simulink model "SIL_model"  (R2020a)
settings: Solver=ode4  StartTime=0.0  StopTime=30  FixedStep=0.001  RelTol=1e-3
InitFcn:
  | Init_control;
values from neighbouring files (symbols this model uses):
  layer1 = double(results{1,1}.layer9)    [load_parameter.m]
  layer2 = double(results{1,1}.layer10)    [load_parameter.m]
  layer3 = double(results{1,1}.layer11)    [load_parameter.m]
  layer4 = double(results{1,1}.layer12)    [load_parameter.m]
  layer5 = double(results{1,1}.layer13)    [load_parameter.m]
  layer6 = double(results{1,1}.layer14)    [load_parameter.m]
  std = sqrt(max(a,0.01))    [load_parameter.m]
undefined symbols (not defined in the file or in its folder): DWORK0, DWORK1, DWORK10, DWORK11, DWORK12, DWORK13, DWORK14, DWORK15, DWORK2, DWORK3, DWORK4, DWORK5, DWORK6, DWORK7, DWORK8, DWORK9, earthRadius, KiPitchAttitude, KiRollAttitude, Kp_RP_ANGLE, MAX_CONTROL_ANGLE_RATE_Y, MAX_CONTROL_ANGLE_RP, ModelInit_RPM, ModelParam_envAltitude, ModelParam_GlobalNoiseGainSwitch, ModelParam_GPSLatLong, ModelParam_motorCr, ModelParam_motorJm, ModelParam_motorMinThr, ModelParam_motorT, ModelParam_motorWb, ModelParam_rotorCm, ModelParam_rotorCt, ModelParam_uavCCm, ModelParam_uavCd, ModelParam_uavDearo, ModelParam_uavJ, ModelParam_uavMass, ModelParam_uavR, ModelParam_uavType, Receive, Send
libraries: aerolibfltsims x4, simulink x2, shared6dof x1, aerolibanimutils x1
(part 2 of 2)

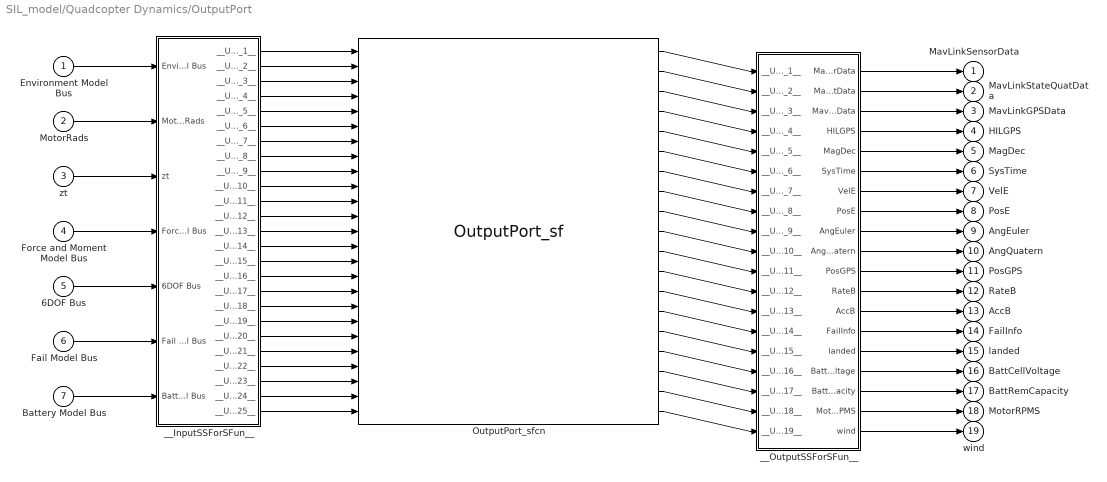
== system SIL_model/Quadcopter Dynamics/OutputPort ==
  Environment Model Bus : Inport
  MotorRads : Inport  Port=2
  zt : Inport  Port=3
  Force and Moment Model Bus : Inport  Port=4
  6DOF Bus : Inport  Port=5
  Fail Model Bus : Inport  Port=6
  Battery Model Bus : Inport  Port=7
  OutputPort_sfcn : S-Function  FunctionName=OutputPort_sf  Parameters=sfcnParam1, sfcnParam2, sfcnParam3  SFunctionModules=""  SFunctionDeploymentMode=off  EnableBusSupport=off  SFcnStateName=DWORK0,DWORK1,DWORK2,DWORK3,DWORK4,DWORK5,DWORK6,DWORK7,DWORK8,DWORK9  mask{rtw_sf_name=OutputPort_sf, showVar=off, sfcnParam1=sfcnParam1, sfcnParam2=sfcnParam2, sfcnParam3=sfcnParam3}
      mask prompts: rtw_sf_name "Simulink:masks:GenSFuncName_MP"; showVar "Simulink:masks:GenSFuncShowModuleList_MP"; sfcnParam1 "ModelParam_GPSLatLong:"; sfcnParam2 "ModelParam_GlobalNoiseGainSwitch:"; sfcnParam3 "ModelParam_envAltitude:"
      mask help: Simulink:masks:GenSFuncDesc_MD
      mask init: same as SIL_model/Quadcopter Dynamics/Battery Model/Battery Model_sfcn
      settings: SFcnIsStateOwnerBlock=on
      settings: CopyFcn=|
      | if ~strcmp(get_param(gcb,'Linkstatus'),'none') && ...
      | ~strcmp(get_param(gcb,'Linkstatus'),'implicit')
      |   set_param(gcb,'LinkStatus','none');
      | end
      mask Help: eval('feval(''rtwprivate'',''rtwhelpview'',''rtw_sfcn_block'')');
      mask Display:
      | port_label('input',1,'PosGPS');
      | port_label('input',2,'gravity');
      | port_label('input',3,'TempC');
      | port_label('input',4,'AirPressure');
      | port_label('input',5,'Rho');
      | port_label('input',6,'Windb');
      | port_label('input',7,'Wind');
      | port_label('input',8,'MotorRads');
      | port_label('input',9,'zt');
      | port_label('input',10,'Fb');
      | port_label('input',11,'Mb');
      | port_label('input',12,'landed');
      | port_label('input',13,'Ve');
      | port_label('input',14,'Xe');
      | port_label('input',15,'Eular(rad)');
      | port_label('input',16,'DCM');
      | port_label('input',17,'Vb');
      | port_label('input',18,'wb');
      | port_label('input',19,'dwb/dt');
      | port_label('input',20,'m');
      | port_label('input',21,'J');
      | port_label('input',22,'dM');
      | port_label('input',23,'PWMOut');
      | port_label('input',24,'cellVol');
      | port_label('input',25,'remCapa');
      | port_label('output',1,'MavLinkSensorData');
      | port_label('output',2,'MavLinkStateQuatData');
      | port_label('output',3,'MavLinkGPSData');
      | port_label('output',4,'HILGPS');
      | port_label('output',5,'MagDec');
      | port_label('output',6,'SysTime');
      | port_label('output',7,'VelE');
      | port_label('output',8,'PosE');
      | port_label('output',9,'AngEuler');
      | port_label('output',10,'AngQuatern');
      | port_label('output',11,'PosGPSb');
      | port_label('output',12,'RateB');
      | port_label('output',13,'AccB');
      | port_label('output',14,'FailInfo');
      | port_label('output',15,'landedb');
      | port_label('output',16,'BattCellVoltage');
      | port_label('output',17,'BattRemCapacity');
      | port_label('output',18,'MotorRPMS');
      | port_label('output',19,'wind');
  __InputSSForSFun__ : Subsystem
  __OutputSSForSFun__ : Subsystem
  MavLinkSensorData : Outport  OutDataTypeStr=Bus: MavLinkSensor  SampleTime=[-1 0]  VectorParamsAs1DForOutWhenUnconnected=off  BusOutputAsStruct=on
  MavLinkStateQuatData : Outport  Port=2  OutDataTypeStr=Bus: MavLinkStateQuat  SampleTime=[-1 0]  VectorParamsAs1DForOutWhenUnconnected=off  BusOutputAsStruct=on
  MavLinkGPSData : Outport  Port=3  OutDataTypeStr=Bus: MavLinkGPS  SampleTime=[-1 0]  VectorParamsAs1DForOutWhenUnconnected=off  BusOutputAsStruct=on
  HILGPS : Outport  Port=4  OutDataTypeStr=Bus: HILGPS  SampleTime=[-1 0]  VectorParamsAs1DForOutWhenUnconnected=off  BusOutputAsStruct=on
  MagDec : Outport  Port=5  VectorParamsAs1DForOutWhenUnconnected=off
  SysTime : Outport  Port=6  VectorParamsAs1DForOutWhenUnconnected=off
  VelE : Outport  Port=7  VectorParamsAs1DForOutWhenUnconnected=off
  PosE : Outport  Port=8  VectorParamsAs1DForOutWhenUnconnected=off
  AngEuler : Outport  Port=9  VectorParamsAs1DForOutWhenUnconnected=off
  AngQuatern : Outport  Port=10  VectorParamsAs1DForOutWhenUnconnected=off
  PosGPS : Outport  Port=11  VectorParamsAs1DForOutWhenUnconnected=off
  RateB : Outport  Port=12  VectorParamsAs1DForOutWhenUnconnected=off
  AccB : Outport  Port=13  VectorParamsAs1DForOutWhenUnconnected=off
  FailInfo : Outport  Port=14  VectorParamsAs1DForOutWhenUnconnected=off
  landed : Outport  Port=15  VectorParamsAs1DForOutWhenUnconnected=off
  BattCellVoltage : Outport  Port=16  VectorParamsAs1DForOutWhenUnconnected=off
  BattRemCapacity : Outport  Port=17  VectorParamsAs1DForOutWhenUnconnected=off
  MotorRPMS : Outport  Port=18  VectorParamsAs1DForOutWhenUnconnected=off
  wind : Outport  Port=19  VectorParamsAs1DForOutWhenUnconnected=off
  wires:
  Environment Model Bus/1 -> __InputSSForSFun__/1(Environment Model Bus)
  MotorRads/1 -> __InputSSForSFun__/2(MotorRads)
  zt/1 -> __InputSSForSFun__/3(zt)
  Force and Moment Model Bus/1 -> __InputSSForSFun__/4(Force and Moment Model Bus)
  6DOF Bus/1 -> __InputSSForSFun__/5(6DOF Bus)
  Fail Model Bus/1 -> __InputSSForSFun__/6(Fail Model Bus)
  Battery Model Bus/1 -> __InputSSForSFun__/7(Battery Model Bus)
  __InputSSForSFun__/1(__UniqueOutportName__1__) -> OutputPort_sfcn/1
  __InputSSForSFun__/2(__UniqueOutportName__2__) -> OutputPort_sfcn/2
  __InputSSForSFun__/3(__UniqueOutportName__3__) -> OutputPort_sfcn/3
  __InputSSForSFun__/4(__UniqueOutportName__4__) -> OutputPort_sfcn/4
  __InputSSForSFun__/5(__UniqueOutportName__5__) -> OutputPort_sfcn/5
  __InputSSForSFun__/6(__UniqueOutportName__6__) -> OutputPort_sfcn/6
  __InputSSForSFun__/7(__UniqueOutportName__7__) -> OutputPort_sfcn/7
  __InputSSForSFun__/8(__UniqueOutportName__8__) -> OutputPort_sfcn/8
  __InputSSForSFun__/9(__UniqueOutportName__9__) -> OutputPort_sfcn/9
  __InputSSForSFun__/10(__UniqueOutportName__10__) -> OutputPort_sfcn/10
  __InputSSForSFun__/11(__UniqueOutportName__11__) -> OutputPort_sfcn/11
  __InputSSForSFun__/12(__UniqueOutportName__12__) -> OutputPort_sfcn/12
  __InputSSForSFun__/13(__UniqueOutportName__13__) -> OutputPort_sfcn/13
  __InputSSForSFun__/14(__UniqueOutportName__14__) -> OutputPort_sfcn/14
  __InputSSForSFun__/15(__UniqueOutportName__15__) -> OutputPort_sfcn/15
  __InputSSForSFun__/16(__UniqueOutportName__16__) -> OutputPort_sfcn/16
  __InputSSForSFun__/17(__UniqueOutportName__17__) -> OutputPort_sfcn/17
  __InputSSForSFun__/18(__UniqueOutportName__18__) -> OutputPort_sfcn/18
  __InputSSForSFun__/19(__UniqueOutportName__19__) -> OutputPort_sfcn/19
  __InputSSForSFun__/20(__UniqueOutportName__20__) -> OutputPort_sfcn/20
  __InputSSForSFun__/21(__UniqueOutportName__21__) -> OutputPort_sfcn/21
  __InputSSForSFun__/22(__UniqueOutportName__22__) -> OutputPort_sfcn/22
  __InputSSForSFun__/23(__UniqueOutportName__23__) -> OutputPort_sfcn/23
  __InputSSForSFun__/24(__UniqueOutportName__24__) -> OutputPort_sfcn/24
  __InputSSForSFun__/25(__UniqueOutportName__25__) -> OutputPort_sfcn/25
  OutputPort_sfcn/1 -> __OutputSSForSFun__/1(__UniqueInportName__1__)
  OutputPort_sfcn/2 -> __OutputSSForSFun__/2(__UniqueInportName__2__)
  OutputPort_sfcn/3 -> __OutputSSForSFun__/3(__UniqueInportName__3__)
  OutputPort_sfcn/4 -> __OutputSSForSFun__/4(__UniqueInportName__4__)
  OutputPort_sfcn/5 -> __OutputSSForSFun__/5(__UniqueInportName__5__)
  OutputPort_sfcn/6 -> __OutputSSForSFun__/6(__UniqueInportName__6__)
  OutputPort_sfcn/7 -> __OutputSSForSFun__/7(__UniqueInportName__7__)
  OutputPort_sfcn/8 -> __OutputSSForSFun__/8(__UniqueInportName__8__)
  OutputPort_sfcn/9 -> __OutputSSForSFun__/9(__UniqueInportName__9__)
  OutputPort_sfcn/10 -> __OutputSSForSFun__/10(__UniqueInportName__10__)
  OutputPort_sfcn/11 -> __OutputSSForSFun__/11(__UniqueInportName__11__)
  OutputPort_sfcn/12 -> __OutputSSForSFun__/12(__UniqueInportName__12__)
  OutputPort_sfcn/13 -> __OutputSSForSFun__/13(__UniqueInportName__13__)
  OutputPort_sfcn/14 -> __OutputSSForSFun__/14(__UniqueInportName__14__)
  OutputPort_sfcn/15 -> __OutputSSForSFun__/15(__UniqueInportName__15__)
  OutputPort_sfcn/16 -> __OutputSSForSFun__/16(__UniqueInportName__16__)
  OutputPort_sfcn/17 -> __OutputSSForSFun__/17(__UniqueInportName__17__)
  OutputPort_sfcn/18 -> __OutputSSForSFun__/18(__UniqueInportName__18__)
  OutputPort_sfcn/19 -> __OutputSSForSFun__/19(__UniqueInportName__19__)
  __OutputSSForSFun__/1(MavLinkSensorData) -> MavLinkSensorData/1
  __OutputSSForSFun__/2(MavLinkStateQuatData) -> MavLinkStateQuatData/1
  __OutputSSForSFun__/3(MavLinkGPSData) -> MavLinkGPSData/1
  __OutputSSForSFun__/4(HILGPS) -> HILGPS/1
  __OutputSSForSFun__/5(MagDec) -> MagDec/1
  __OutputSSForSFun__/6(SysTime) -> SysTime/1
  __OutputSSForSFun__/7(VelE) -> VelE/1
  __OutputSSForSFun__/8(PosE) -> PosE/1
  __OutputSSForSFun__/9(AngEuler) -> AngEuler/1
  __OutputSSForSFun__/10(AngQuatern) -> AngQuatern/1
  __OutputSSForSFun__/11(PosGPS) -> PosGPS/1
  __OutputSSForSFun__/12(RateB) -> RateB/1
  __OutputSSForSFun__/13(AccB) -> AccB/1
  __OutputSSForSFun__/14(FailInfo) -> FailInfo/1
  __OutputSSForSFun__/15(landed) -> landed/1
  __OutputSSForSFun__/16(BattCellVoltage) -> BattCellVoltage/1
  __OutputSSForSFun__/17(BattRemCapacity) -> BattRemCapacity/1
  __OutputSSForSFun__/18(MotorRPMS) -> MotorRPMS/1
  __OutputSSForSFun__/19(wind) -> wind/1

== system SIL_model/Quadcopter Dynamics/Separation of float Data1 ==
  note: 小数部分
  float_Data : Inport
  Add2 : Sum  Inputs=+-
  Integer Uint : Constant  Value=IntUint
  Math Function1 : Math  Operator=mod  SignedPower=on  SaturateOnIntegerOverflow=on
  Integer_Part : Outport  VectorParamsAs1DForOutWhenUnconnected=off
  decimalt_Part : Outport  Port=2  VectorParamsAs1DForOutWhenUnconnected=off
  wires:
  Math Function1/1 -> decimalt_Part/1, Add2/2
  Integer Uint/1 -> Math Function1/2
  Add2/1 -> Integer_Part/1
  float_Data/1 -> Math Function1/1, Add2/1

== system SIL_model/Quadcopter Dynamics/Battery Model/__InputSSForSFun__ ==
  PWMin : Inport
  __UniqueOutportName__1__ : Outport  VectorParamsAs1DForOutWhenUnconnected=off
  wires:
  PWMin/1 -> __UniqueOutportName__1__/1

== system SIL_model/Quadcopter Dynamics/Battery Model/__OutputSSForSFun__ ==
  __UniqueInportName__1__ : Inport
  __UniqueInportName__2__ : Inport  Port=2
  __UniqueInportName__3__ : Inport  Port=3
  Mux1 : BusCreator  Inputs=3
  Battery Model Bus : Outport  VectorParamsAs1DForOutWhenUnconnected=off
  wires:
  __UniqueInportName__1__/1 -> Mux1/1  "PWMOut"
  __UniqueInportName__2__/1 -> Mux1/2  "cellVol"
  __UniqueInportName__3__/1 -> Mux1/3  "remCapa"
  Mux1/1 -> Battery Model Bus/1

== system SIL_model/Quadcopter Dynamics/Environment Model/__InputSSForSFun__ ==
  6DOF Bus : Inport
  temporaryBusSelectName_1 : BusSelector  OutputSignals=Ve,Xe,Eular(rad),DCM,Vb,wb,dwb/dt
  __UniqueOutportName__1__ : Outport  VectorParamsAs1DForOutWhenUnconnected=off
  __UniqueOutportName__2__ : Outport  Port=2  VectorParamsAs1DForOutWhenUnconnected=off
  __UniqueOutportName__3__ : Outport  Port=3  VectorParamsAs1DForOutWhenUnconnected=off
  __UniqueOutportName__4__ : Outport  Port=4  VectorParamsAs1DForOutWhenUnconnected=off
  __UniqueOutportName__5__ : Outport  Port=5  VectorParamsAs1DForOutWhenUnconnected=off
  __UniqueOutportName__6__ : Outport  Port=6  VectorParamsAs1DForOutWhenUnconnected=off
  __UniqueOutportName__7__ : Outport  Port=7  VectorParamsAs1DForOutWhenUnconnected=off
  wires:
  6DOF Bus/1 -> temporaryBusSelectName_1/1
  temporaryBusSelectName_1/1 -> __UniqueOutportName__1__/1  "<Ve>"
  temporaryBusSelectName_1/2 -> __UniqueOutportName__2__/1  "<Xe>"
  temporaryBusSelectName_1/3 -> __UniqueOutportName__3__/1  "<Eular(rad)>"
  temporaryBusSelectName_1/4 -> __UniqueOutportName__4__/1  "<DCM>"
  temporaryBusSelectName_1/5 -> __UniqueOutportName__5__/1  "<Vb>"
  temporaryBusSelectName_1/6 -> __UniqueOutportName__6__/1  "<wb>"
  temporaryBusSelectName_1/7 -> __UniqueOutportName__7__/1  "<dwb/dt>"

== system SIL_model/Quadcopter Dynamics/Environment Model/__OutputSSForSFun__ ==
  __UniqueInportName__1__ : Inport
  __UniqueInportName__2__ : Inport  Port=2
  __UniqueInportName__3__ : Inport  Port=3
  __UniqueInportName__4__ : Inport  Port=4
  __UniqueInportName__5__ : Inport  Port=5
  __UniqueInportName__6__ : Inport  Port=6
  __UniqueInportName__7__ : Inport  Port=7
  Mux1 : BusCreator  Inputs=7
  Environment Model Bus : Outport  VectorParamsAs1DForOutWhenUnconnected=off
  wires:
  __UniqueInportName__1__/1 -> Mux1/1  "PosGPS"
  __UniqueInportName__2__/1 -> Mux1/2  "gravity"
  __UniqueInportName__3__/1 -> Mux1/3  "TempC"
  __UniqueInportName__4__/1 -> Mux1/4  "AirPressure"
  __UniqueInportName__5__/1 -> Mux1/5  "Rho"
  __UniqueInportName__6__/1 -> Mux1/6  "Windb"
  __UniqueInportName__7__/1 -> Mux1/7  "Wind"
  Mux1/1 -> Environment Model Bus/1

== system SIL_model/Quadcopter Dynamics/Fail Model/__InputSSForSFun__ ==
  6DOF Bus : Inport
  temporaryBusSelectName_1 : BusSelector  OutputSignals=Ve,Xe,Eular(rad),DCM,Vb,wb,dwb/dt
  __UniqueOutportName__1__ : Outport  VectorParamsAs1DForOutWhenUnconnected=off
  __UniqueOutportName__2__ : Outport  Port=2  VectorParamsAs1DForOutWhenUnconnected=off
  __UniqueOutportName__3__ : Outport  Port=3  VectorParamsAs1DForOutWhenUnconnected=off
  __UniqueOutportName__4__ : Outport  Port=4  VectorParamsAs1DForOutWhenUnconnected=off
  __UniqueOutportName__5__ : Outport  Port=5  VectorParamsAs1DForOutWhenUnconnected=off
  __UniqueOutportName__6__ : Outport  Port=6  VectorParamsAs1DForOutWhenUnconnected=off
  __UniqueOutportName__7__ : Outport  Port=7  VectorParamsAs1DForOutWhenUnconnected=off
  wires:
  6DOF Bus/1 -> temporaryBusSelectName_1/1
  temporaryBusSelectName_1/1 -> __UniqueOutportName__1__/1  "<Ve>"
  temporaryBusSelectName_1/2 -> __UniqueOutportName__2__/1  "<Xe>"
  temporaryBusSelectName_1/3 -> __UniqueOutportName__3__/1  "<Eular(rad)>"
  temporaryBusSelectName_1/4 -> __UniqueOutportName__4__/1  "<DCM>"
  temporaryBusSelectName_1/5 -> __UniqueOutportName__5__/1  "<Vb>"
  temporaryBusSelectName_1/6 -> __UniqueOutportName__6__/1  "<wb>"
  temporaryBusSelectName_1/7 -> __UniqueOutportName__7__/1  "<dwb/dt>"

== system SIL_model/Quadcopter Dynamics/Fail Model/__OutputSSForSFun__ ==
  __UniqueInportName__1__ : Inport
  __UniqueInportName__2__ : Inport  Port=2
  __UniqueInportName__3__ : Inport  Port=3
  Mux1 : BusCreator  Inputs=3
  Fail Model Bus : Outport  VectorParamsAs1DForOutWhenUnconnected=off
  wires:
  __UniqueInportName__1__/1 -> Mux1/1  "m"
  __UniqueInportName__2__/1 -> Mux1/2  "J"
  __UniqueInportName__3__/1 -> Mux1/3  "dM"
  Mux1/1 -> Fail Model Bus/1

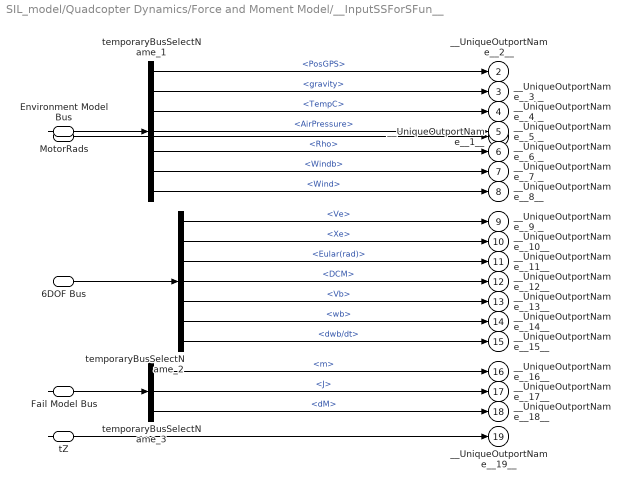
== system SIL_model/Quadcopter Dynamics/Force and Moment Model/__InputSSForSFun__ ==
  MotorRads : Inport
  Environment Model Bus : Inport  Port=2
  6DOF Bus : Inport  Port=3
  Fail Model Bus : Inport  Port=4
  "tZ " : Inport  Port=5
  temporaryBusSelectName_1 : BusSelector  OutputSignals=PosGPS,gravity,TempC,AirPressure,Rho,Windb,Wind
  temporaryBusSelectName_2 : BusSelector  OutputSignals=Ve,Xe,Eular(rad),DCM,Vb,wb,dwb/dt
  temporaryBusSelectName_3 : BusSelector  OutputSignals=m,J,dM
  __UniqueOutportName__1__ : Outport  VectorParamsAs1DForOutWhenUnconnected=off
  __UniqueOutportName__2__ : Outport  Port=2  VectorParamsAs1DForOutWhenUnconnected=off
  __UniqueOutportName__3__ : Outport  Port=3  VectorParamsAs1DForOutWhenUnconnected=off
  __UniqueOutportName__4__ : Outport  Port=4  VectorParamsAs1DForOutWhenUnconnected=off
  __UniqueOutportName__5__ : Outport  Port=5  VectorParamsAs1DForOutWhenUnconnected=off
  __UniqueOutportName__6__ : Outport  Port=6  VectorParamsAs1DForOutWhenUnconnected=off
  __UniqueOutportName__7__ : Outport  Port=7  VectorParamsAs1DForOutWhenUnconnected=off
  __UniqueOutportName__8__ : Outport  Port=8  VectorParamsAs1DForOutWhenUnconnected=off
  __UniqueOutportName__9__ : Outport  Port=9  VectorParamsAs1DForOutWhenUnconnected=off
  __UniqueOutportName__10__ : Outport  Port=10  VectorParamsAs1DForOutWhenUnconnected=off
  __UniqueOutportName__11__ : Outport  Port=11  VectorParamsAs1DForOutWhenUnconnected=off
  __UniqueOutportName__12__ : Outport  Port=12  VectorParamsAs1DForOutWhenUnconnected=off
  __UniqueOutportName__13__ : Outport  Port=13  VectorParamsAs1DForOutWhenUnconnected=off
  __UniqueOutportName__14__ : Outport  Port=14  VectorParamsAs1DForOutWhenUnconnected=off
  __UniqueOutportName__15__ : Outport  Port=15  VectorParamsAs1DForOutWhenUnconnected=off
  __UniqueOutportName__16__ : Outport  Port=16  VectorParamsAs1DForOutWhenUnconnected=off
  __UniqueOutportName__17__ : Outport  Port=17  VectorParamsAs1DForOutWhenUnconnected=off
  __UniqueOutportName__18__ : Outport  Port=18  VectorParamsAs1DForOutWhenUnconnected=off
  __UniqueOutportName__19__ : Outport  Port=19  VectorParamsAs1DForOutWhenUnconnected=off
  wires:
  Environment Model Bus/1 -> temporaryBusSelectName_1/1
  6DOF Bus/1 -> temporaryBusSelectName_2/1
  Fail Model Bus/1 -> temporaryBusSelectName_3/1
  MotorRads/1 -> __UniqueOutportName__1__/1
  temporaryBusSelectName_1/1 -> __UniqueOutportName__2__/1  "<PosGPS>"
  temporaryBusSelectName_1/2 -> __UniqueOutportName__3__/1  "<gravity>"
  temporaryBusSelectName_1/3 -> __UniqueOutportName__4__/1  "<TempC>"
  temporaryBusSelectName_1/4 -> __UniqueOutportName__5__/1  "<AirPressure>"
  temporaryBusSelectName_1/5 -> __UniqueOutportName__6__/1  "<Rho>"
  temporaryBusSelectName_1/6 -> __UniqueOutportName__7__/1  "<Windb>"
  temporaryBusSelectName_1/7 -> __UniqueOutportName__8__/1  "<Wind>"
  temporaryBusSelectName_2/1 -> __UniqueOutportName__9__/1  "<Ve>"
  temporaryBusSelectName_2/2 -> __UniqueOutportName__10__/1  "<Xe>"
  temporaryBusSelectName_2/3 -> __UniqueOutportName__11__/1  "<Eular(rad)>"
  temporaryBusSelectName_2/4 -> __UniqueOutportName__12__/1  "<DCM>"
  temporaryBusSelectName_2/5 -> __UniqueOutportName__13__/1  "<Vb>"
  temporaryBusSelectName_2/6 -> __UniqueOutportName__14__/1  "<wb>"
  temporaryBusSelectName_2/7 -> __UniqueOutportName__15__/1  "<dwb/dt>"
  temporaryBusSelectName_3/1 -> __UniqueOutportName__16__/1  "<m>"
  temporaryBusSelectName_3/2 -> __UniqueOutportName__17__/1  "<J>"
  temporaryBusSelectName_3/3 -> __UniqueOutportName__18__/1  "<dM>"
  "tZ "/1 -> __UniqueOutportName__19__/1

== system SIL_model/Quadcopter Dynamics/Force and Moment Model/__OutputSSForSFun__ ==
  __UniqueInportName__1__ : Inport
  __UniqueInportName__2__ : Inport  Port=2
  __UniqueInportName__3__ : Inport  Port=3
  Mux1 : BusCreator  Inputs=3
  Force and Moment Model Bus : Outport  VectorParamsAs1DForOutWhenUnconnected=off
  wires:
  __UniqueInportName__1__/1 -> Mux1/1  "Fb"
  __UniqueInportName__2__/1 -> Mux1/2  "Mb"
  __UniqueInportName__3__/1 -> Mux1/3  "landed"
  Mux1/1 -> Force and Moment Model Bus/1

== system SIL_model/Quadcopter Dynamics/Motor Model/__InputSSForSFun__ ==
  Battery Model Bus : Inport
  temporaryBusSelectName_1 : BusSelector  OutputSignals=PWMOut,cellVol,remCapa
  __UniqueOutportName__1__ : Outport  VectorParamsAs1DForOutWhenUnconnected=off
  __UniqueOutportName__2__ : Outport  Port=2  VectorParamsAs1DForOutWhenUnconnected=off
  __UniqueOutportName__3__ : Outport  Port=3  VectorParamsAs1DForOutWhenUnconnected=off
  wires:
  Battery Model Bus/1 -> temporaryBusSelectName_1/1
  temporaryBusSelectName_1/1 -> __UniqueOutportName__1__/1  "<PWMOut>"
  temporaryBusSelectName_1/2 -> __UniqueOutportName__2__/1  "<cellVol>"
  temporaryBusSelectName_1/3 -> __UniqueOutportName__3__/1  "<remCapa>"

== system SIL_model/Quadcopter Dynamics/Motor Model/__OutputSSForSFun__ ==
  __UniqueInportName__1__ : Inport
  MotorRads : Outport  VectorParamsAs1DForOutWhenUnconnected=off
  wires:
  __UniqueInportName__1__/1 -> MotorRads/1  "y"

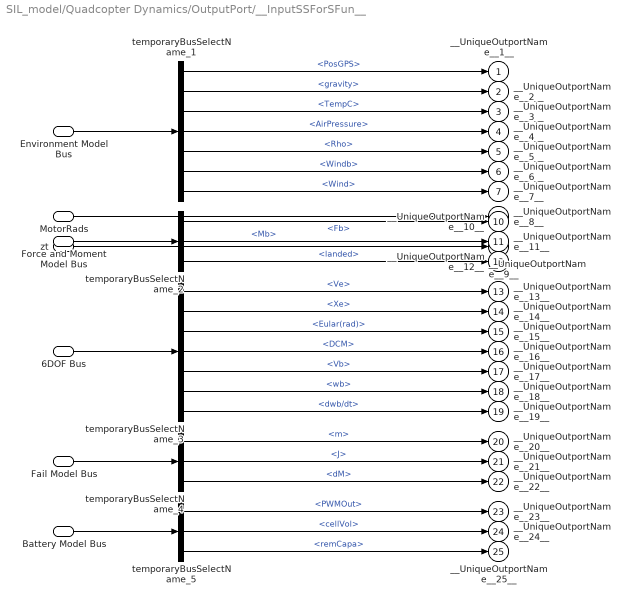
== system SIL_model/Quadcopter Dynamics/OutputPort/__InputSSForSFun__ ==
  Environment Model Bus : Inport
  MotorRads : Inport  Port=2
  zt : Inport  Port=3
  Force and Moment Model Bus : Inport  Port=4
  6DOF Bus : Inport  Port=5
  Fail Model Bus : Inport  Port=6
  Battery Model Bus : Inport  Port=7
  temporaryBusSelectName_1 : BusSelector  OutputSignals=PosGPS,gravity,TempC,AirPressure,Rho,Windb,Wind
  temporaryBusSelectName_2 : BusSelector  OutputSignals=Fb,Mb,landed
  temporaryBusSelectName_3 : BusSelector  OutputSignals=Ve,Xe,Eular(rad),DCM,Vb,wb,dwb/dt
  temporaryBusSelectName_4 : BusSelector  OutputSignals=m,J,dM
  temporaryBusSelectName_5 : BusSelector  OutputSignals=PWMOut,cellVol,remCapa
  __UniqueOutportName__1__ : Outport  VectorParamsAs1DForOutWhenUnconnected=off
  __UniqueOutportName__2__ : Outport  Port=2  VectorParamsAs1DForOutWhenUnconnected=off
  __UniqueOutportName__3__ : Outport  Port=3  VectorParamsAs1DForOutWhenUnconnected=off
  __UniqueOutportName__4__ : Outport  Port=4  VectorParamsAs1DForOutWhenUnconnected=off
  __UniqueOutportName__5__ : Outport  Port=5  VectorParamsAs1DForOutWhenUnconnected=off
  __UniqueOutportName__6__ : Outport  Port=6  VectorParamsAs1DForOutWhenUnconnected=off
  __UniqueOutportName__7__ : Outport  Port=7  VectorParamsAs1DForOutWhenUnconnected=off
  __UniqueOutportName__8__ : Outport  Port=8  VectorParamsAs1DForOutWhenUnconnected=off
  __UniqueOutportName__9__ : Outport  Port=9  VectorParamsAs1DForOutWhenUnconnected=off
  __UniqueOutportName__10__ : Outport  Port=10  VectorParamsAs1DForOutWhenUnconnected=off
  __UniqueOutportName__11__ : Outport  Port=11  VectorParamsAs1DForOutWhenUnconnected=off
  __UniqueOutportName__12__ : Outport  Port=12  VectorParamsAs1DForOutWhenUnconnected=off
  __UniqueOutportName__13__ : Outport  Port=13  VectorParamsAs1DForOutWhenUnconnected=off
  __UniqueOutportName__14__ : Outport  Port=14  VectorParamsAs1DForOutWhenUnconnected=off
  __UniqueOutportName__15__ : Outport  Port=15  VectorParamsAs1DForOutWhenUnconnected=off
  __UniqueOutportName__16__ : Outport  Port=16  VectorParamsAs1DForOutWhenUnconnected=off
  __UniqueOutportName__17__ : Outport  Port=17  VectorParamsAs1DForOutWhenUnconnected=off
  __UniqueOutportName__18__ : Outport  Port=18  VectorParamsAs1DForOutWhenUnconnected=off
  __UniqueOutportName__19__ : Outport  Port=19  VectorParamsAs1DForOutWhenUnconnected=off
  __UniqueOutportName__20__ : Outport  Port=20  VectorParamsAs1DForOutWhenUnconnected=off
  __UniqueOutportName__21__ : Outport  Port=21  VectorParamsAs1DForOutWhenUnconnected=off
  __UniqueOutportName__22__ : Outport  Port=22  VectorParamsAs1DForOutWhenUnconnected=off
  __UniqueOutportName__23__ : Outport  Port=23  VectorParamsAs1DForOutWhenUnconnected=off
  __UniqueOutportName__24__ : Outport  Port=24  VectorParamsAs1DForOutWhenUnconnected=off
  __UniqueOutportName__25__ : Outport  Port=25  VectorParamsAs1DForOutWhenUnconnected=off
  wires:
  Environment Model Bus/1 -> temporaryBusSelectName_1/1
  Force and Moment Model Bus/1 -> temporaryBusSelectName_2/1
  6DOF Bus/1 -> temporaryBusSelectName_3/1
  Fail Model Bus/1 -> temporaryBusSelectName_4/1
  Battery Model Bus/1 -> temporaryBusSelectName_5/1
  temporaryBusSelectName_1/1 -> __UniqueOutportName__1__/1  "<PosGPS>"
  temporaryBusSelectName_1/2 -> __UniqueOutportName__2__/1  "<gravity>"
  temporaryBusSelectName_1/3 -> __UniqueOutportName__3__/1  "<TempC>"
  temporaryBusSelectName_1/4 -> __UniqueOutportName__4__/1  "<AirPressure>"
  temporaryBusSelectName_1/5 -> __UniqueOutportName__5__/1  "<Rho>"
  temporaryBusSelectName_1/6 -> __UniqueOutportName__6__/1  "<Windb>"
  temporaryBusSelectName_1/7 -> __UniqueOutportName__7__/1  "<Wind>"
  MotorRads/1 -> __UniqueOutportName__8__/1
  zt/1 -> __UniqueOutportName__9__/1
  temporaryBusSelectName_2/1 -> __UniqueOutportName__10__/1  "<Fb>"
  temporaryBusSelectName_2/2 -> __UniqueOutportName__11__/1  "<Mb>"
  temporaryBusSelectName_2/3 -> __UniqueOutportName__12__/1  "<landed>"
  temporaryBusSelectName_3/1 -> __UniqueOutportName__13__/1  "<Ve>"
  temporaryBusSelectName_3/2 -> __UniqueOutportName__14__/1  "<Xe>"
  temporaryBusSelectName_3/3 -> __UniqueOutportName__15__/1  "<Eular(rad)>"
  temporaryBusSelectName_3/4 -> __UniqueOutportName__16__/1  "<DCM>"
  temporaryBusSelectName_3/5 -> __UniqueOutportName__17__/1  "<Vb>"
  temporaryBusSelectName_3/6 -> __UniqueOutportName__18__/1  "<wb>"
  temporaryBusSelectName_3/7 -> __UniqueOutportName__19__/1  "<dwb/dt>"
  temporaryBusSelectName_4/1 -> __UniqueOutportName__20__/1  "<m>"
  temporaryBusSelectName_4/2 -> __UniqueOutportName__21__/1  "<J>"
  temporaryBusSelectName_4/3 -> __UniqueOutportName__22__/1  "<dM>"
  temporaryBusSelectName_5/1 -> __UniqueOutportName__23__/1  "<PWMOut>"
  temporaryBusSelectName_5/2 -> __UniqueOutportName__24__/1  "<cellVol>"
  temporaryBusSelectName_5/3 -> __UniqueOutportName__25__/1  "<remCapa>"

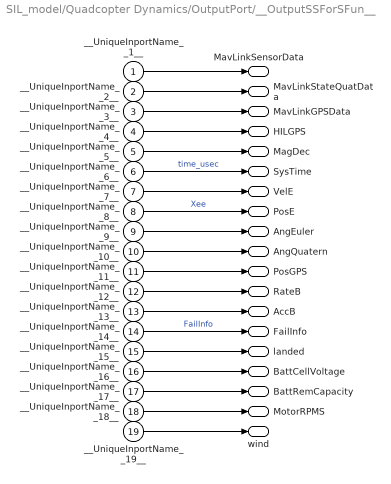
== system SIL_model/Quadcopter Dynamics/OutputPort/__OutputSSForSFun__ ==
  __UniqueInportName__1__ : Inport
  __UniqueInportName__2__ : Inport  Port=2
  __UniqueInportName__3__ : Inport  Port=3
  __UniqueInportName__4__ : Inport  Port=4
  __UniqueInportName__5__ : Inport  Port=5
  __UniqueInportName__6__ : Inport  Port=6
  __UniqueInportName__7__ : Inport  Port=7
  __UniqueInportName__8__ : Inport  Port=8
  __UniqueInportName__9__ : Inport  Port=9
  __UniqueInportName__10__ : Inport  Port=10
  __UniqueInportName__11__ : Inport  Port=11
  __UniqueInportName__12__ : Inport  Port=12
  __UniqueInportName__13__ : Inport  Port=13
  __UniqueInportName__14__ : Inport  Port=14
  __UniqueInportName__15__ : Inport  Port=15
  __UniqueInportName__16__ : Inport  Port=16
  __UniqueInportName__17__ : Inport  Port=17
  __UniqueInportName__18__ : Inport  Port=18
  __UniqueInportName__19__ : Inport  Port=19
  MavLinkSensorData : Outport  OutDataTypeStr=Bus: MavLinkSensor  SampleTime=[-1 0]  VectorParamsAs1DForOutWhenUnconnected=off  BusOutputAsStruct=on
  MavLinkStateQuatData : Outport  Port=2  OutDataTypeStr=Bus: MavLinkStateQuat  SampleTime=[-1 0]  VectorParamsAs1DForOutWhenUnconnected=off  BusOutputAsStruct=on
  MavLinkGPSData : Outport  Port=3  OutDataTypeStr=Bus: MavLinkGPS  SampleTime=[-1 0]  VectorParamsAs1DForOutWhenUnconnected=off  BusOutputAsStruct=on
  HILGPS : Outport  Port=4  OutDataTypeStr=Bus: HILGPS  SampleTime=[-1 0]  VectorParamsAs1DForOutWhenUnconnected=off  BusOutputAsStruct=on
  MagDec : Outport  Port=5  VectorParamsAs1DForOutWhenUnconnected=off
  SysTime : Outport  Port=6  VectorParamsAs1DForOutWhenUnconnected=off
  VelE : Outport  Port=7  VectorParamsAs1DForOutWhenUnconnected=off
  PosE : Outport  Port=8  VectorParamsAs1DForOutWhenUnconnected=off
  AngEuler : Outport  Port=9  VectorParamsAs1DForOutWhenUnconnected=off
  AngQuatern : Outport  Port=10  VectorParamsAs1DForOutWhenUnconnected=off
  PosGPS : Outport  Port=11  VectorParamsAs1DForOutWhenUnconnected=off
  RateB : Outport  Port=12  VectorParamsAs1DForOutWhenUnconnected=off
  AccB : Outport  Port=13  VectorParamsAs1DForOutWhenUnconnected=off
  FailInfo : Outport  Port=14  VectorParamsAs1DForOutWhenUnconnected=off
  landed : Outport  Port=15  VectorParamsAs1DForOutWhenUnconnected=off
  BattCellVoltage : Outport  Port=16  VectorParamsAs1DForOutWhenUnconnected=off
  BattRemCapacity : Outport  Port=17  VectorParamsAs1DForOutWhenUnconnected=off
  MotorRPMS : Outport  Port=18  VectorParamsAs1DForOutWhenUnconnected=off
  wind : Outport  Port=19  VectorParamsAs1DForOutWhenUnconnected=off
  wires:
  __UniqueInportName__1__/1 -> MavLinkSensorData/1
  __UniqueInportName__2__/1 -> MavLinkStateQuatData/1
  __UniqueInportName__3__/1 -> MavLinkGPSData/1
  __UniqueInportName__4__/1 -> HILGPS/1
  __UniqueInportName__5__/1 -> MagDec/1
  __UniqueInportName__6__/1 -> SysTime/1  "time_usec"
  __UniqueInportName__7__/1 -> VelE/1
  __UniqueInportName__8__/1 -> PosE/1  "Xee"
  __UniqueInportName__9__/1 -> AngEuler/1
  __UniqueInportName__10__/1 -> AngQuatern/1
  __UniqueInportName__11__/1 -> PosGPS/1
  __UniqueInportName__12__/1 -> RateB/1
  __UniqueInportName__13__/1 -> AccB/1
  __UniqueInportName__14__/1 -> FailInfo/1  "FailInfo"
  __UniqueInportName__15__/1 -> landed/1
  __UniqueInportName__16__/1 -> BattCellVoltage/1
  __UniqueInportName__17__/1 -> BattRemCapacity/1
  __UniqueInportName__18__/1 -> MotorRPMS/1
  __UniqueInportName__19__/1 -> wind/1

== matlab function SIL_model/Control System1/InputConditioning/MATLAB Function ==
  data: u input; y output
function y = fcn(u)
%将遥控输入的范围控制在1100~1900，同时设置一个死区，死区大小为±deadZone
RCMin = 1100;
RCMax = 1900;
deadZoneRate = 0.05;
deadZone = deadZoneRate*(RCMax-RCMin);
%限幅
if(u < RCMin)
    u = RCMin;
elseif(u > RCMax)
    u = RCMax;
end
%死区
 if(u > 1500+deadZone)
    y = u;
 elseif(u < 1500-deadZone)
     y = u;
 else
     y = 1500;
 end
     
 end

== matlab function SIL_model/Control System1/InputConditioning/MATLAB Function1 ==
  data: u input; y output
function y = fcn(u)
%将遥控输入的范围控制在1100~1900，同时设置一个死区，死区大小为±deadZone
RCMin = 1100;
RCMax = 1900;
deadZoneRate = 0.05;
deadZone = deadZoneRate*(RCMax-RCMin);
%限幅
if(u < RCMin)
    u = RCMin;
elseif(u > RCMax)
    u = RCMax;
end
%死区
 if(u > 1500+deadZone)
    y = u;
 elseif(u < 1500-deadZone)
     y = u;
 else
     y = 1500;
 end
     
 end

== matlab function SIL_model/Control System1/InputConditioning/MATLAB Function2 ==
  data: u input; y output
function y = fcn(u)
%将遥控输入的范围控制在1100~1900，同时设置一个死区，死区大小为±deadZone
RCMin = 1100;
RCMax = 1900;
deadZoneRate = 0.05;
deadZone = deadZoneRate*(RCMax-RCMin);
%限幅
if(u < RCMin)
    u = RCMin;
elseif(u > RCMax)
    u = RCMax;
end
%死区
 if(u > 1500+deadZone)
    y = u;
 elseif(u < 1500-deadZone)
     y = u;
 else
     y = 1500;
 end
     
 end

== matlab function SIL_model/Control System1/pwm_out1 ==
  data: Roll input; M1 output; Pitch input; Yaw input; d_roll input; M2 output; M3 output; M4 output; d_pitch input; d_yaw input; thrust input; mean input; std input; layer1 input; layer2 input; layer3 input; layer4 input; layer5 input; layer6 input
function [M1, M2, M3, M4] = motor_mixer(Roll, Pitch, Yaw,d_roll, d_pitch, d_yaw, thrust, mean, std,layer1,layer2,layer3,layer4,layer5,layer6)


ob = [Roll, Pitch, Yaw,d_roll, d_pitch, d_yaw];
ob = (ob-reshape(mean,1,6))./reshape(std,1,6);
ob = max(ob,[-5.0,-5.0,-5.0,-5.0,-5.0,-5.0]);
ob = min(ob, [5.0,5.0,5.0,5.0,5.0,5.0]);
layer_1 = tanh(ob * layer1 + reshape(layer2, 1, 64));
layer_2 = tanh(layer_1 * layer3 + reshape(layer4, 1, 64));
output = layer_2 * layer5 + reshape(layer6,1,4);

u = output;
for i = 1:4
    if output(i)>1
        output(i)=1;
    end
    if output(i)<-1
        output(i) = -1;
    end
    output(i) = (output(i)+1)/2;
end
%O1 = u(1);
%O2 = u(2);
%O3 = u(3);
%O4 = u(4);
pwm = 1500*output + 1000*thrust + 1000;
M1 = ( pwm(1)) ;
M2 = ( pwm(4)) ;              
M3 = ( pwm(3)) ;
M4 = ( pwm(2)) ;


% Quad XROLL （根据QP里面的叉字形结构的文字）
% M1 = ((Pitch+ Yaw)+Thrust-Roll) * 1000 + idle_PWM;
 %M2 = ((Pitch - Yaw)+Thrust+Roll) * 1000 + idle_PWM;
 %M3 = ((Roll +Yaw) + Thrust-Pitch) * 1000 + idle_PWM;
 %M4 = ((-Roll - Pitch-Yaw) + Thrust) * 1000 + idle_PWM;
% M5 = 1000;
% M6 = 1000;
% M7 = 1000;
% M8 = 1000;
%qp上实际的输出
%M1 = (Thrust+Pitch-Roll+Yaw) * 1000 + idle_PWM;
 %M2 = (Thrust-Pitch +Roll+Yaw) * 1000 + idle_PWM;
 %M3 = ( Thrust+Roll+Pitch-Yaw) * 1000 + idle_PWM;
 %M4 = (Thrust-Roll- Pitch -Yaw) * 1000 + idle_PWM;
% Quad +
 %M1 = ((Pitch - Yaw) * Thrust / 2 + Thrust) * 1000 + idle_PWM;
 %M2 = ((-Roll + Yaw) * Thrust / 2 + Thrust) * 1000 + idle_PWM;
% M3 = ((-Pitch - Yaw) * Thrust / 2 + Thrust) * 1000 + idle_PWM;
 %M4 = ((Roll + Yaw) * Thrust / 2 + Thrust) * 1000 + idle_PWM;
% M5 = 1000;
% M6 = 1000;
% M7 = 1000;
% M8 = 1000;

% Hex X
% M1 = ((Pitch + Roll / 2 - Yaw) * Thrust / 2 + Thrust) * 1000 + idle_PWM;
% M2 = ((Pitch - Roll / 2 + Yaw) * Thrust / 2 + Thrust) * 1000 + idle_PWM;
% M3 = ((-Roll - Yaw) * Thrust / 2 + Thrust) * 1000 + idle_PWM;
% M4 = ((-Pitch - Roll / 2 + Yaw) * Thrust / 2 + Thrust) * 1000 + idle_PWM;
% M5 = ((-Pitch + Roll / 2 - Yaw) * Thrust / 2 + Thrust) * 1000 + idle_PWM;
% M6 = ((Roll + Yaw) * Thrust / 2 + Thrust) * 1000 + idle_PWM;
% M7 = 1000;
% M8 = 1000;

% Hex X (From Adam)
%M1 = uint16(single(((-Roll - Yaw) * Thrust / 3 + Thrust) * single(1000))) + idle_PWM;
%M2 = uint16(single(((Roll + Yaw) * Thrust / 3 + Thrust) * single(1000))) + idle_PWM;
%M3 = uint16(single(((Pitch + (Roll / 2) - Yaw) * Thrust / 3 + Thrust) * single(1000))) + idle_PWM;
%M4 = uint16(single(((-Pitch - (Roll / 2) + Yaw) * Thrust / 3 + Thrust) * single(1000))) + idle_PWM;
%M5 = uint16(single(((Pitch - (Roll / 2) + Yaw) * Thrust / 3 + Thrust) * single(1000))) + idle_PWM;
%M6 = uint16(single(((-Pitch + (Roll / 2) - Yaw) * Thrust / 3 + Thrust) * single(1000))) + idle_PWM;

% Hex X (Version 2)
% Roll/Yaw
% M1 = ((-Roll - Yaw) * Thrust / 2 + Thrust) * 1000 + idle_PWM;
% M2 = ((Roll + Yaw) * Thrust / 2 + Thrust) * 1000 + idle_PWM;
% % + Pitch/Roll
% M6 = ((Pitch + Roll / 2 - Yaw) * Thrust / 2 + Thrust) * 1000 + idle_PWM;
% M4 = ((Pitch - Roll / 2 + Yaw) * Thrust / 2 + Thrust) * 1000 + idle_PWM;
% % - Pitch/Roll
% M5 = ((-Pitch - Roll / 2 + Yaw) * Thrust / 2 + Thrust) * 1000 + idle_PWM;
% M3 = ((-Pitch + Roll / 2 - Yaw) * Thrust / 2 + Thrust) * 1000 + idle_PWM;

== matlab function SIL_model/Control System1/InputConditioning/MATLAB Function3 ==
  data: u input; y output
function y = fcn(u)
%将遥控输入的范围控制在1100~1900，同时设置一个死区，死区大小为±deadZone
RCMin = 1100;
RCMax = 1900;
deadZoneRate = 0.05;
deadZone = deadZoneRate*(RCMax-RCMin);
%限幅
if(u < RCMin)
    u = RCMin;
elseif(u > RCMax)
    u = RCMax;
end
%死区
 if(u > 1500+deadZone)
    y = u;
 elseif(u < 1500-deadZone)
     y = u;
 else
     y = 1500;
 end
     
 end
